simulink model "BT_Observer1"  (R2019a)
settings: Solver=FixedStepAuto  StartTime=0.0  StopTime=10.0  FixedStep=0.01  RelTol=1e-3
values from neighbouring files (symbols this model uses):
  A = [0 1 0; 0 -4 -0.03;0 0.6 -10]    [observer_DC.m]
  B = [0;0;8.237]    [observer_DC.m]
  C = [1 0 0]    [observer_DC.m]
  L = [46; 653.982; 12688.267]    [observer_DC.m]
settings Model: Creator=Thien  LastModifiedBy=ASUS
settings DataIOCC: ReturnWorkspaceOutputs=off
settings DebuggingCC: ArithmeticOperatorsInVariantConditions=warning
settings SFSimCC: SimUseLocalCustomCode=off
settings RTWCC: RTWUseLocalCustomCode=off
settings CodeAppCC: StateflowObjectComments=on

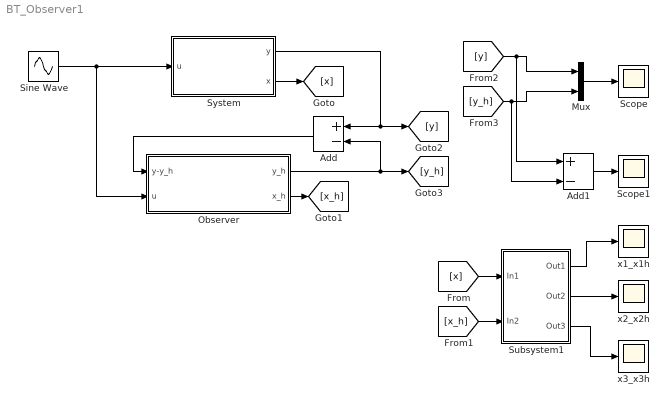
== system BT_Observer1 ==
  Add : Sum  Inputs=+-
  Add1 : Sum  Inputs=+-
  Mux : Mux  Inputs=2
  Observer : Subsystem
  Scope : Scope
  Scope1 : Scope
  Sine Wave : Sin  Amplitude=2  Frequency=2*pi*0.1  SampleTime=0
  Subsystem1 : Subsystem
  System : Subsystem
  x1_x1h : Scope
  x2_x2h : Scope
  x3_x3h : Scope
  wires:
  Add/1 -> Observer/1(y-y_h)
  Observer/1(y_h) -> [y_h], Add/2
  System/1(y) -> Add/1, [y]
  Sine Wave/1 -> Observer/2(u), System/1(u)
  System/2(x) -> [x]
  Observer/2(x_h) -> [x_h]
  Mux/1 -> Scope/1
  [y] -> Add1/1, Mux/1
  [y_h] -> Add1/2, Mux/2
  Add1/1 -> Scope1/1
  [x] -> Subsystem1/1(In1)
  [x_h] -> Subsystem1/2(In2)
  Subsystem1/1(Out1) -> x1_x1h/1
  Subsystem1/2(Out2) -> x2_x2h/1
  Subsystem1/3(Out3) -> x3_x3h/1

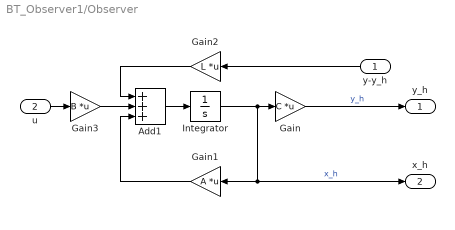
== system BT_Observer1/Observer ==
  y-y_h : Inport
  u : Inport  Port=2
  Add1 : Sum  Inputs=+++
  Gain : Gain  Gain=C  Multiplication=Matrix(K*u) (u vector)
  Gain1 : Gain  Gain=A  Multiplication=Matrix(K*u) (u vector)
  Gain2 : Gain  Gain=L  Multiplication=Matrix(K*u) (u vector)
  Gain3 : Gain  Gain=B  Multiplication=Matrix(K*u) (u vector)
  Integrator : Integrator  InitialCondition=[0 0 0]'
  y_h : Outport
  x_h : Outport  Port=2
  wires:
  Gain/1 -> y_h/1  "y_h"
  Gain2/1 -> Add1/1
  u/1 -> Gain3/1
  Integrator/1 -> x_h/1, Gain1/1, Gain/1  "x_h"
  y-y_h/1 -> Gain2/1
  Gain1/1 -> Add1/3
  Gain3/1 -> Add1/2
  Add1/1 -> Integrator/1

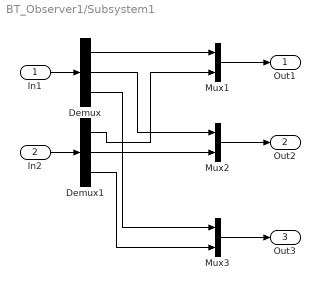
== system BT_Observer1/Subsystem1 ==
  In1 : Inport
  In2 : Inport  Port=2
  Demux : Demux  Outputs=3
  Demux1 : Demux  Outputs=3
  Mux1 : Mux  Inputs=2
  Mux2 : Mux  Inputs=2
  Mux3 : Mux  Inputs=2
  Out1 : Outport
  Out2 : Outport  Port=2
  Out3 : Outport  Port=3
  wires:
  Mux1/1 -> Out1/1
  Demux1/3 -> Mux3/2
  Demux/2 -> Mux2/1
  Mux3/1 -> Out3/1
  Demux1/1 -> Mux1/2
  Mux2/1 -> Out2/1
  Demux/1 -> Mux1/1
  Demux1/2 -> Mux2/2
  In2/1 -> Demux1/1
  In1/1 -> Demux/1
  Demux/3 -> Mux3/1

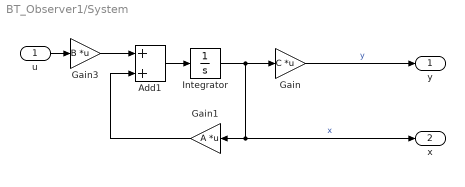
== system BT_Observer1/System ==
  u : Inport
  Add1 : Sum
  Gain : Gain  Gain=C  Multiplication=Matrix(K*u) (u vector)
  Gain1 : Gain  Gain=A  Multiplication=Matrix(K*u) (u vector)
  Gain3 : Gain  Gain=B  Multiplication=Matrix(K*u) (u vector)
  Integrator : Integrator  InitialCondition=[1 0 0]'
  y : Outport
  x : Outport  Port=2
  wires:
  Gain1/1 -> Add1/2
  Add1/1 -> Integrator/1
  Integrator/1 -> Gain/1, x/1, Gain1/1  "x"
  Gain/1 -> y/1  "y"
  Gain3/1 -> Add1/1
  u/1 -> Gain3/1
